simulink model "Rider_Controls_ControlHarness"  (R2014b)
settings: configuration reference "Embedded_Configuration" (kept outside this file)
PostLoadFcn:
  | load('Embedded_Config.mat')
model workspace: external: MAT-File C:\Users\Sean\Desktop\Buckeye Current\MagicSimNode\Rider_Controls.mat (data not in the file)
undefined symbols (not defined in the file or in its folder): canChannel, sigbuilder_block
libraries: canlib x10, canmsglib x8, dspswit3 x2, simulink x1, realtime_pacer_lib x1, dspsigattribs x1
settings Model: Creator=The MathWorks Inc.  LastModifiedBy=Sean

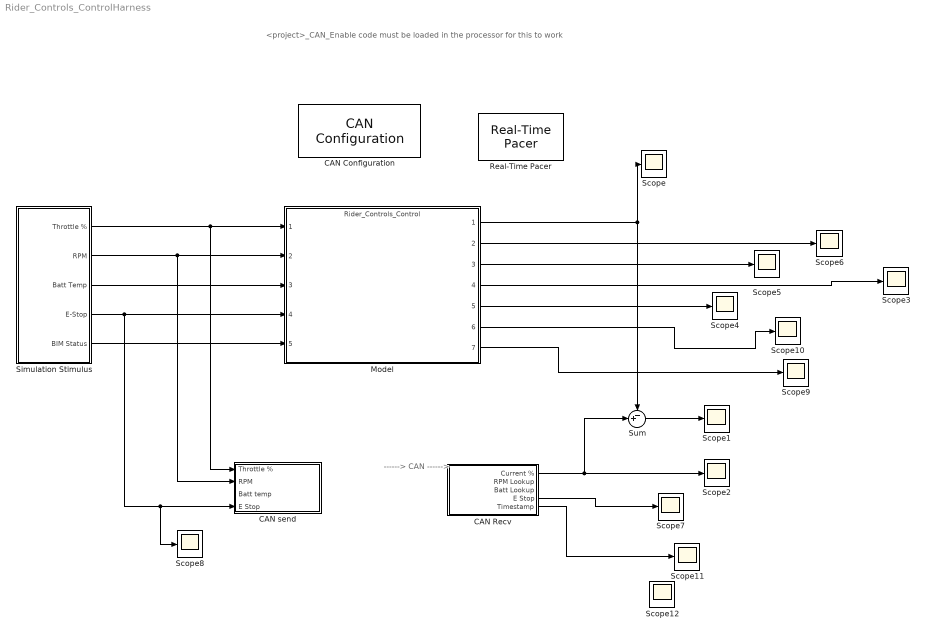
== system Rider_Controls_ControlHarness ==
  note: <project>_CAN_Enable code must be loaded
      | in the processor for this to work
  note: ------> CAN ------>
  CAN Configuration : canlib/CAN Configuration  BlockHandle=3197.0009  DeviceMenu=Kvaser Virtual 1 (Channel 1)  Device=Kvaser Eagle 1 (Channel 1)  ObjConstructor=canChannel('Kvaser', 'Eagle 1', 1)  BusSpeed=500000  EnableBitParameters=off  SJW=1  TSEG1=4  TSEG2=3  NSamples=1  AckMode=Normal
  CAN Recv : Subsystem
  CAN send : Subsystem
  Model : ModelReference  ModelNameDialog=Rider_Controls_Control.slx  SimulationMode=Normal  ModelReferenceVersion=1.163  CopyOfModelName=Rider_Controls_Control.slx  DefaultDataLogging=on
  Real-Time Pacer : realtime_pacer_lib/Real-Time Pacer  simTimePerRealTime=1
  Scope{,1..12} (13 alike) : Scope
      Scope settings: YMin=-0.2  YMax=1.2
      Scope10 settings: SaveName=ScopeData10
      Scope11 settings: TimeRange=20  SaveName=ScopeData11
      Scope12 settings: TimeRange=10  YMin=0  YMax=4  SaveName=ScopeData12
      Scope2 settings: TimeRange=10  SaveName=ScopeData2
      Scope3 settings: SaveName=ScopeData3
      Scope4 settings: SaveName=ScopeData4
      Scope5 settings: YMin=-0.2  YMax=1.2  SaveName=ScopeData5
      Scope6 settings: YMin=-0.2  YMax=1.2  SaveName=ScopeData6
      Scope7 settings: TimeRange=10  SaveName=ScopeData7
      Scope8 settings: TimeRange=10  SaveName=ScopeData8
      Scope9 settings: SaveName=ScopeData9
  Simulation Stimulus : Subsystem
  Sum : Sum  Inputs=-+|
  wires:
  CAN Recv/1(Current %) -> Sum/2, Scope2/1
  Sum/1 -> Scope1/1
  Simulation Stimulus/1("Throttle % ") -> CAN send/1(Throttle %), Model/1
  Simulation Stimulus/2(RPM) -> CAN send/2(RPM), Model/2
  Simulation Stimulus/3(Batt Temp) -> Model/3
  Model/1 -> Sum/1, Scope/1
  Model/4 -> Scope3/1
  Model/5 -> Scope4/1
  Model/2 -> Scope6/1
  Model/3 -> Scope5/1
  Simulation Stimulus/4(E-Stop) -> Scope8/1, CAN send/4(E Stop), Model/4
  CAN Recv/4(E Stop) -> Scope7/1
  Model/7 -> Scope9/1
  Simulation Stimulus/5(BIM Status) -> Model/5
  Model/6 -> Scope10/1
  CAN Recv/5(Timestamp) -> Scope11/1
  ? -> Scope12/1

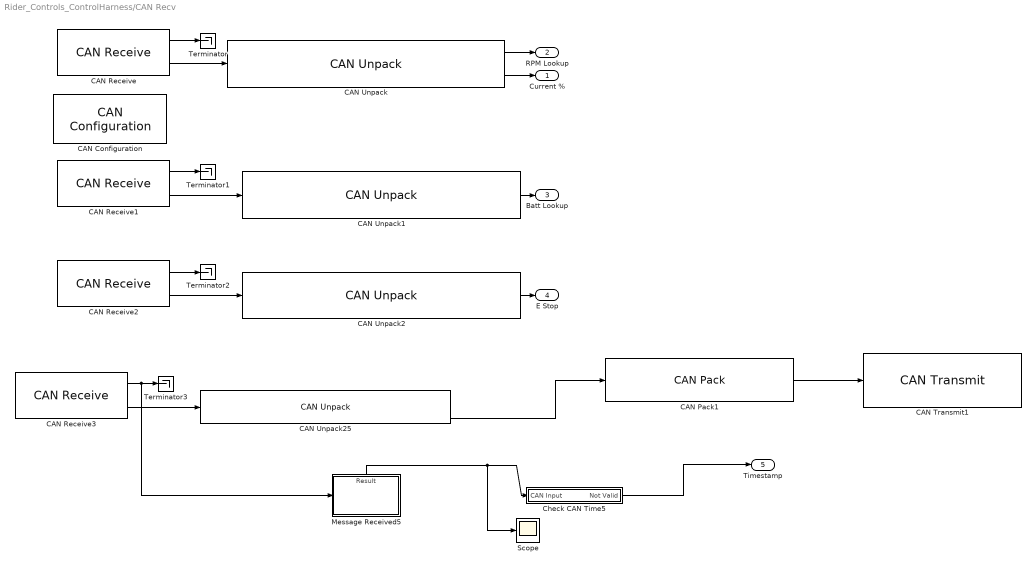
== system Rider_Controls_ControlHarness/CAN Recv ==
  CAN Configuration : canlib/CAN Configuration  BlockHandle=3204.0009  DeviceMenu=Kvaser Virtual 1 (Channel 1)  Device=Kvaser Virtual 1 (Channel 1)  ObjConstructor=canChannel('Kvaser', 'Virtual 1', 1)  BusSpeed=500000  EnableBitParameters=off  SJW=1  TSEG1=4  TSEG2=3  NSamples=1  AckMode=Normal
  CAN Pack1 : canmsglib/CAN Pack  CANdbFile=C:\Users\Nathan\Desktop\Git\EmbeddedCoderC2000\Rider_Controls\Rider_Controls_Debug.dbc  MsgList=Control_Input3  MsgName=Control_Input3  MsgIDType=Standard (11-bit identifier)  MsgIdentifier=2  MsgLength=8  SignalInfo=Batt_Temp$0$32$1$3$1$0$1$0$-10000$10000$#  NSignals=1  StartBits=str2num('[int32(0)]')  SignalSizes=str2num('[int32(32)]')  ByteOrders=str2num('[int32(1)]')  DataTypes=str2num('[int32(3)]')  MultiplexTypes=str2num('[int32(1)]')  MultiplexValues=str2num('[double(0)]')  Factors=str2num('[double(1)]')  Offsets=str2num('[double(0)]')  Minimums=str2num('[double(-10000)]')  Maximums=str2num('[double(10000)]')  Remote=off
      settings: DataFormat=CANdb specified signals
  CAN Receive : canlib/CAN Receive  BlockHandle=3206.0009  DeviceMenu=Kvaser Virtual 1 (Channel 1)  Device=Kvaser Eagle 1 (Channel 1)  ObjConstructor=canChannel('Kvaser', 'Eagle 1', 1)  EnableStandardIDsFilter=off  StandardIDs=1  EnableExtendedIDsFilter=off  ExtendedIDs=0  SampleTime=.01  MsgsPerTimestep=all  StdIDsCombo=Allow only  ExtIDsCombo=Block all  InternalFilterUpdateStatus=on
  CAN Receive1 : canlib/CAN Receive  BlockHandle=3207.0009  DeviceMenu=Kvaser Virtual 1 (Channel 1)  Device=Kvaser Eagle 1 (Channel 1)  ObjConstructor=canChannel('Kvaser', 'Eagle 1', 1)  EnableStandardIDsFilter=off  StandardIDs=3  EnableExtendedIDsFilter=off  ExtendedIDs=0  SampleTime=.01  MsgsPerTimestep=all  StdIDsCombo=Allow only  ExtIDsCombo=Block all  InternalFilterUpdateStatus=on
  CAN Receive2 : canlib/CAN Receive  BlockHandle=4510.0004  DeviceMenu=Kvaser Virtual 1 (Channel 1)  Device=Kvaser Eagle 1 (Channel 1)  ObjConstructor=canChannel('Kvaser', 'Eagle 1', 1)  EnableStandardIDsFilter=off  StandardIDs=5  EnableExtendedIDsFilter=off  ExtendedIDs=0  SampleTime=.01  MsgsPerTimestep=all  StdIDsCombo=Allow only  ExtIDsCombo=Block all  InternalFilterUpdateStatus=on
  CAN Receive3 : canlib/CAN Receive  BlockHandle=4511.0004  DeviceMenu=Kvaser Eagle 1 (Channel 1)  Device=Kvaser Eagle 1 (Channel 1)  ObjConstructor=canChannel('Kvaser', 'Eagle 1', 1)  EnableStandardIDsFilter=off  StandardIDs=831  EnableExtendedIDsFilter=off  ExtendedIDs=0  SampleTime=.5  MsgsPerTimestep=all  StdIDsCombo=Allow only  ExtIDsCombo=Block all  InternalFilterUpdateStatus=on
  CAN Transmit1 : canlib/CAN Transmit  BlockHandle=4512.0004  DeviceMenu=Kvaser Virtual 1 (Channel 1)  Device=Kvaser Eagle 1 (Channel 1)  ObjConstructor=canChannel('Kvaser', 'Eagle 1', 1)  EnablePeriodicTransmit=on  MessagePeriod=.01
  CAN Unpack : canmsglib/CAN Unpack  CANdbFile=C:\Users\Nathan\Desktop\Git\EmbeddedCoderC2000\Rider_Controls\Rider_Controls_Debug.dbc  MsgList=Control_Ouput  MsgName=Control_Ouput  MsgIDType=Standard (11-bit identifier)  MsgIdentifier=1  MsgLength=8  SignalInfo=Lookup$32$32$1$3$1$0$1$0$-10000$10000$#Motor_Current_percent$0$32$1$3$1$0$1$0$-1000$1000$#  NSignals=2  IDPort=off  TimestampPort=off  ErrorPort=off  RemotePort=off  LengthPort=off  StatusPort=off  StartBits=str2num('[int32(32);int32(0)]')  SignalSizes=str2num('[int32(32);int32(32)]')  ByteOrders=str2num('[int32(1);int32(1)]')  DataTypes=str2num('[int32(3);int32(3)]')  MultiplexTypes=str2num('[int32(1);int32(1)]')  MultiplexValues=str2num('[double(0);double(0)]')  Factors=str2num('[double(1);double(1)]')  Offsets=str2num('[double(0);double(0)]')  Minimums=str2num('[double(-10000);double(-1000)]')  Maximums=str2num('[double(10000);double(1000)]')
      settings: DataFormat=CANdb specified signals
  CAN Unpack1 : canmsglib/CAN Unpack  CANdbFile=C:\Users\Nathan\Desktop\Git\EmbeddedCoderC2000\Rider_Controls\Rider_Controls_Debug.dbc  MsgList=Control_Output3  MsgName=Control_Output3  MsgIDType=Standard (11-bit identifier)  MsgIdentifier=3  MsgLength=8  SignalInfo=Batt_Lookup$0$32$1$3$1$0$1$0$-1000$10000$#  NSignals=1  IDPort=off  TimestampPort=off  ErrorPort=off  RemotePort=off  LengthPort=off  StatusPort=off  StartBits=str2num('[int32(0)]')  SignalSizes=str2num('[int32(32)]')  ByteOrders=str2num('[int32(1)]')  DataTypes=str2num('[int32(3)]')  MultiplexTypes=str2num('[int32(1)]')  MultiplexValues=str2num('[double(0)]')  Factors=str2num('[double(1)]')  Offsets=str2num('[double(0)]')  Minimums=str2num('[double(-1000)]')  Maximums=str2num('[double(10000)]')
      settings: DataFormat=CANdb specified signals
  CAN Unpack2 : canmsglib/CAN Unpack  CANdbFile=C:\Users\Nathan\Desktop\Git\EmbeddedCoderC2000\Rider_Controls\Rider_Controls_Debug.dbc  MsgList=Control_Output4  MsgName=Control_Output4  MsgIDType=Standard (11-bit identifier)  MsgIdentifier=5  MsgLength=8  SignalInfo=EStop$0$32$1$3$1$0$1$0$-Inf$Inf$#  NSignals=1  IDPort=off  TimestampPort=off  ErrorPort=off  RemotePort=off  LengthPort=off  StatusPort=off  StartBits=str2num('[int32(0)]')  SignalSizes=str2num('[int32(32)]')  ByteOrders=str2num('[int32(1)]')  DataTypes=str2num('[int32(3)]')  MultiplexTypes=str2num('[int32(1)]')  MultiplexValues=str2num('[double(0)]')  Factors=str2num('[double(1)]')  Offsets=str2num('[double(0)]')  Minimums=str2num('[double(-Inf)]')  Maximums=str2num('[double(Inf)]')
      settings: DataFormat=CANdb specified signals
  CAN Unpack25 : canmsglib/CAN Unpack  CANdbFile=C:\Users\Sean\Desktop\Buckeye Current\Databases\RW3.dbc  MsgList=CellTemp20  MsgName=CellTemp20  MsgIDType=Standard (11-bit identifier)  MsgIdentifier=831  MsgLength=8  SignalInfo=CellTemp39$0$32$1$3$1$0$1$0$-Inf$Inf$#CellTemp40$32$32$1$3$1$0$1$0$-Inf$Inf$#  NSignals=2  IDPort=off  TimestampPort=on  ErrorPort=off  RemotePort=off  LengthPort=off  StatusPort=off  StartBits=str2num('[int32(0);int32(32)]')  SignalSizes=str2num('[int32(32);int32(32)]')  ByteOrders=str2num('[int32(1);int32(1)]')  DataTypes=str2num('[int32(3);int32(3)]')  MultiplexTypes=str2num('[int32(1);int32(1)]')  MultiplexValues=str2num('[double(0);double(0)]')  Factors=str2num('[double(1);double(1)]')  Offsets=str2num('[double(0);double(0)]')  Minimums=str2num('[double(-Inf);double(-Inf)]')  Maximums=str2num('[double(Inf);double(Inf)]')
      settings: DataFormat=CANdb specified signals
  Check CAN Time5 : Subsystem
  Message Received5 : Subsystem  TreatAsAtomicUnit=on
  Scope : Scope
      settings: YMin=0  YMax=20  SaveName=ScopeData14
  Terminator{,1..3} (4 alike) : Terminator
  Current % : Outport
  RPM Lookup : Outport  Port=2
  Batt Lookup : Outport  Port=3
  E Stop : Outport  Port=4
  Timestamp : Outport  Port=5
  wires:
  CAN Receive/1 -> Terminator/1
  CAN Receive/2 -> CAN Unpack/1
  CAN Unpack/2 -> Current %/1
  CAN Unpack/1 -> RPM Lookup/1
  CAN Receive1/1 -> Terminator1/1
  CAN Receive1/2 -> CAN Unpack1/1
  CAN Unpack1/1 -> Batt Lookup/1
  CAN Receive2/1 -> Terminator2/1
  CAN Receive2/2 -> CAN Unpack2/1
  CAN Unpack2/1 -> E Stop/1
  CAN Receive3/2 -> CAN Unpack25/1
  CAN Receive3/1 -> Message Received5/Trigger, Terminator3/1
  CAN Unpack25/3 -> CAN Pack1/1
  CAN Pack1/1 -> CAN Transmit1/1
  Message Received5/1(Result) -> Scope/1, Check CAN Time5/1(CAN Input)
  Check CAN Time5/1(Not Valid) -> Timestamp/1

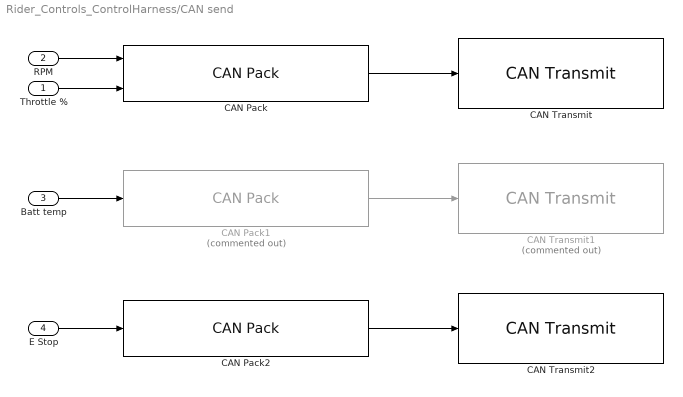
== system Rider_Controls_ControlHarness/CAN send ==
  Throttle % : Inport  OutDataTypeStr=single
  RPM : Inport  Port=2  OutDataTypeStr=single
  Batt temp : Inport  Port=3  OutDataTypeStr=single
  E Stop : Inport  Port=4
  CAN Pack : canmsglib/CAN Pack  CANdbFile=C:\Users\Nathan\Desktop\Git\EmbeddedCoderC2000\Rider_Controls\Rider_Controls_Debug.dbc  MsgList=Control_Input  MsgName=Control_Input12  MsgIDType=Standard (11-bit identifier)  MsgIdentifier=0  MsgLength=8  SignalInfo=RPM$32$32$1$3$1$0$1$0$-100000$100000$#Throttle$0$32$1$3$1$0$1$0$-1000$1000$#  NSignals=2  StartBits=str2num('[int32(32);int32(0)]')  SignalSizes=str2num('[int32(32);int32(32)]')  ByteOrders=str2num('[int32(1);int32(1)]')  DataTypes=str2num('[int32(3);int32(3)]')  MultiplexTypes=str2num('[int32(1);int32(1)]')  MultiplexValues=str2num('[double(0);double(0)]')  Factors=str2num('[double(1);double(1)]')  Offsets=str2num('[double(0);double(0)]')  Minimums=str2num('[double(-100000);double(-1000)]')  Maximums=str2num('[double(100000);double(1000)]')  Remote=off
      settings: DataFormat=CANdb specified signals
  CAN Pack1 : canmsglib/CAN Pack  Commented=on  CANdbFile=C:\Users\Nathan\Desktop\Git\EmbeddedCoderC2000\Rider_Controls\Rider_Controls_Debug.dbc  MsgList=Control_Input3  MsgName=Control_Input3  MsgIDType=Standard (11-bit identifier)  MsgIdentifier=2  MsgLength=8  SignalInfo=Batt_Temp$0$32$1$3$1$0$1$0$-10000$10000$#  NSignals=1  StartBits=str2num('[int32(0)]')  SignalSizes=str2num('[int32(32)]')  ByteOrders=str2num('[int32(1)]')  DataTypes=str2num('[int32(3)]')  MultiplexTypes=str2num('[int32(1)]')  MultiplexValues=str2num('[double(0)]')  Factors=str2num('[double(1)]')  Offsets=str2num('[double(0)]')  Minimums=str2num('[double(-10000)]')  Maximums=str2num('[double(10000)]')  Remote=off
      settings: DataFormat=CANdb specified signals
  CAN Pack2 : canmsglib/CAN Pack  CANdbFile=C:\Users\Nathan\Desktop\Git\EmbeddedCoderC2000\Rider_Controls\Rider_Controls_Debug.dbc  MsgList=Control_Input4  MsgName=Control_Input4  MsgIDType=Standard (11-bit identifier)  MsgIdentifier=4  MsgLength=8  SignalInfo=EStop$0$32$1$2$1$0$1$0$-Inf$Inf$#  NSignals=1  StartBits=str2num('[int32(0)]')  SignalSizes=str2num('[int32(32)]')  ByteOrders=str2num('[int32(1)]')  DataTypes=str2num('[int32(2)]')  MultiplexTypes=str2num('[int32(1)]')  MultiplexValues=str2num('[double(0)]')  Factors=str2num('[double(1)]')  Offsets=str2num('[double(0)]')  Minimums=str2num('[double(-Inf)]')  Maximums=str2num('[double(Inf)]')  Remote=off
      settings: DataFormat=CANdb specified signals
  CAN Transmit : canlib/CAN Transmit  BlockHandle=4565.0001  DeviceMenu=Kvaser Virtual 1 (Channel 1)  Device=Kvaser Eagle 1 (Channel 1)  ObjConstructor=canChannel('Kvaser', 'Eagle 1', 1)  EnablePeriodicTransmit=on  MessagePeriod=.01
  CAN Transmit1 : canlib/CAN Transmit  Commented=on  BlockHandle=4566.0001  DeviceMenu=Kvaser Virtual 1 (Channel 1)  Device=Kvaser Eagle 1 (Channel 1)  ObjConstructor=canChannel('Kvaser', 'Eagle 1', 1)  EnablePeriodicTransmit=on  MessagePeriod=.01
  CAN Transmit2 : canlib/CAN Transmit  BlockHandle=4567.0001  DeviceMenu=Kvaser Virtual 1 (Channel 1)  Device=Kvaser Eagle 1 (Channel 1)  ObjConstructor=canChannel('Kvaser', 'Eagle 1', 1)  EnablePeriodicTransmit=on  MessagePeriod=.01
  wires:
  CAN Pack/1 -> CAN Transmit/1
  RPM/1 -> CAN Pack/1
  Throttle %/1 -> CAN Pack/2
  Batt temp/1 -> CAN Pack1/1
  CAN Pack1/1 -> CAN Transmit1/1
  E Stop/1 -> CAN Pack2/1
  CAN Pack2/1 -> CAN Transmit2/1

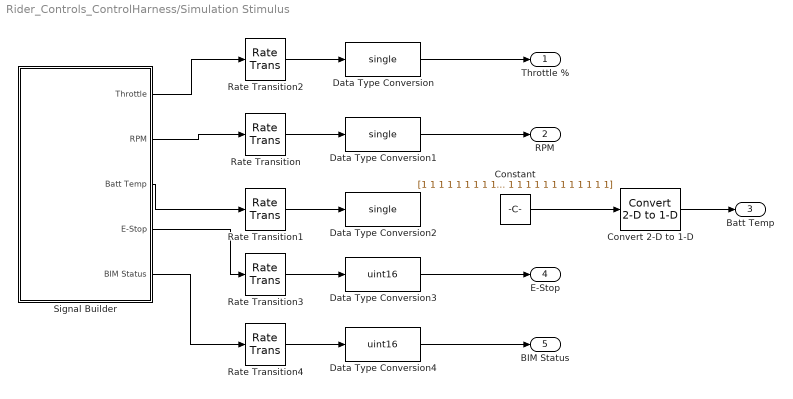
== system Rider_Controls_ControlHarness/Simulation Stimulus ==
  Constant : Constant  Value=[1 1 1 1 1 1 1 1 1 1 1 1 1 1 1 1 1 1 1 1 1 1 1 1 1 1 1 1 1 1 1 1 1 1 1 1 1 1 1 1]  VectorParams1D=off  OutDataTypeStr=single
  Convert 2-D to 1-D : dspsigattribs/Convert 2-D to 1-D
  Data Type Conversion : DataTypeConversion  OutDataTypeStr=single  RndMeth=Simplest
  Data Type Conversion1 : DataTypeConversion  OutDataTypeStr=single  RndMeth=Simplest
  Data Type Conversion2 : DataTypeConversion  OutDataTypeStr=single  RndMeth=Simplest
  Data Type Conversion3 : DataTypeConversion  OutDataTypeStr=uint16  RndMeth=Simplest
  Data Type Conversion4 : DataTypeConversion  OutDataTypeStr=uint16  RndMeth=Simplest
  Rate Transition{,1..4} (5 alike) : RateTransition  OutPortSampleTime=.01
  Signal Builder : Subsystem  Tag=STV Subsys  LoadFcn=sigbuilder_block('load');  StartFcn=sigbuilder_block('start');  StopFcn=sigbuilder_block('stop');  ClipboardFcn=sigbuilder_block('clipboard');  mask(Sigbuilder block){}
      mask help: Simulink:masks:SigbuilderBlock_MD
      mask init:
      | if ~strcmp(get_param(bdroot(gcbh),'SimulationStatus'),'stopped') tuvar = sigbuilder_block('maskInit'); end
      settings: CopyFcn=sigbuilder_block('copy');  DeleteFcn=sigbuilder_block('delete');  ModelCloseFcn=sigbuilder_block('modelClose');  PreSaveFcn=sigbuilder_block('preSave');  PauseFcn=sigbuilder_block('pause');  ContinueFcn=sigbuilder_block('continue');  NameChangeFcn=sigbuilder_block('namechange');  OpenFcn=sigbuilder_block('open',[437.6 199.2 550.4 400 ]);  CloseFcn=sigbuilder_block('close');
      mask Display: plot(0, 0, 100, 100,[2, 2, 32, 32, 2], [68, 8, 8, 68, 68],[32, 2], [38, 38], [32, 19, 2],[53, 60, 44], [32, 17, 17, 2],[16, 16, 31, 31]);txt = getActiveGroup(gcbh);text(2, 100, txt,'verticalAlignment', 'top');
  "Throttle % " : Outport  OutDataTypeStr=single
  RPM : Outport  Port=2  OutDataTypeStr=single
  Batt Temp : Outport  Port=3  OutDataTypeStr=single
  E-Stop : Outport  Port=4
  BIM Status : Outport  Port=5
  wires:
  Rate Transition/1 -> Data Type Conversion1/1
  Signal Builder/2(RPM) -> Rate Transition/1
  Signal Builder/3(Batt Temp) -> Rate Transition1/1
  Rate Transition1/1 -> Data Type Conversion2/1
  Rate Transition2/1 -> Data Type Conversion/1
  Data Type Conversion/1 -> "Throttle % "/1
  Data Type Conversion1/1 -> RPM/1
  Signal Builder/1(Throttle) -> Rate Transition2/1
  Signal Builder/4(E-Stop) -> Rate Transition3/1
  Rate Transition3/1 -> Data Type Conversion3/1
  Data Type Conversion3/1 -> E-Stop/1
  Signal Builder/5(BIM Status) -> Rate Transition4/1
  Rate Transition4/1 -> Data Type Conversion4/1
  Data Type Conversion4/1 -> BIM Status/1
  Constant/1 -> Convert 2-D to 1-D/1
  Convert 2-D to 1-D/1 -> Batt Temp/1

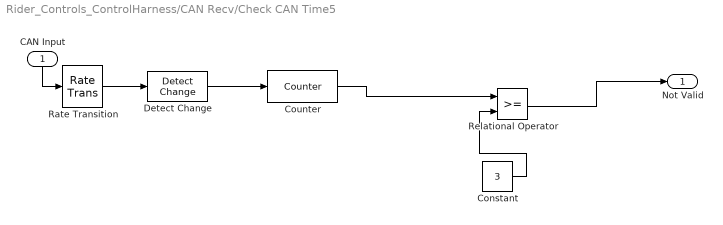
== system Rider_Controls_ControlHarness/CAN Recv/Check CAN Time5 ==
  CAN Input : Inport
  Constant : Constant  Value=3
  Counter : dspswit3/Counter  Direction=Up  CountEvent=Free running  CounterSize=16 bits  MaxCount=255  InitialCount=0  Output=Count  HitValue=1  ResetInput=on  SamplesPerFrame=1  Ts=1  CntDtype=uint16  HitDtype=Logical
  Detect Change : simulink/Logic and Bit Operations/Detect Change  vinit=0  InputProcessing=Inherited  OutDataTypeStr=boolean
  Rate Transition : RateTransition  X0=1  OutPortSampleTime=1
  Relational Operator : RelationalOperator  OutDataTypeStr=boolean
  Not Valid : Outport
  wires:
  CAN Input/1 -> Rate Transition/1
  Relational Operator/1 -> Not Valid/1
  Counter/1 -> Relational Operator/1
  Constant/1 -> Relational Operator/2
  Rate Transition/1 -> Detect Change/1
  Detect Change/1 -> Counter/1

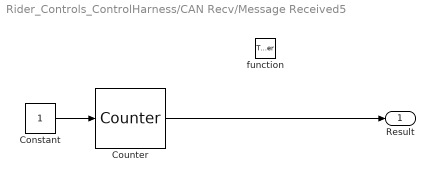
== system Rider_Controls_ControlHarness/CAN Recv/Message Received5 ==
  function : TriggerPort  TriggerType=function-call
  Constant : Constant
  Counter : dspswit3/Counter  Direction=Up  CountEvent=Non-zero sample  CounterSize=16 bits  MaxCount=255  InitialCount=0  Output=Count  HitValue=32  ResetInput=off  SamplesPerFrame=1  Ts=-1  CntDtype=uint16  HitDtype=Logical
  Result : Outport  OutputWhenDisabled=reset  InitialOutput=0
  wires:
  Counter/1 -> Result/1
  Constant/1 -> Counter/1

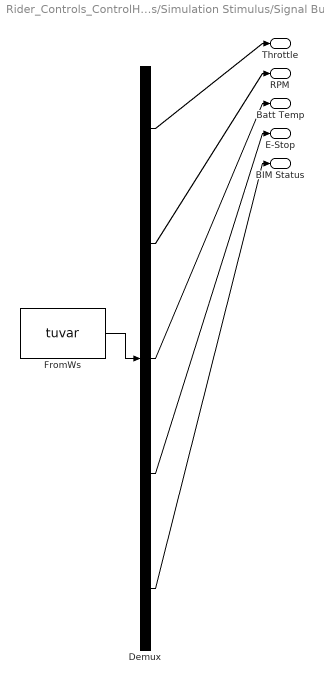
== system Rider_Controls_ControlHarness/Simulation Stimulus/Signal Builder ==
  Demux : Demux  Tag=STV Demux  Outputs=5
  FromWs : FromWorkspace  Tag=STV FromWs  VariableName=tuvar  SampleTime=0
      SigBuilderData=|
      | common.afterFinalStr = 'Extrapolate'
      | common.sampleTime = 0
      | dataSet.timeRange = [0 10]
      | dataSet.name = 'Group 1'
      | sbobj.Groups.Name = 'Group 1'
      | sbobj.Groups.Signals(1).Name = 'Throttle'
      | sbobj.Groups.Signals(1).XData = [0 3.7 3.7 7.26 7.26 10]
      | sbobj.Groups.Signals(1).YData = [0.81 0.81 0.26 0.26 0.11 0.11]
      | sbobj.Groups.Signals(2).Name = 'RPM'
      | sbobj.Groups.Signals(2).XData = [0 3 6.02 10]
      | sbobj.Groups.Signals(2).YData = [0 0 0 4000]
      | sbobj.Groups.Signals(3).Name = 'Batt Temp'
      | sbobj.Groups.Signals(3).XData = [0 3 6 6 10]
      | sbobj.Groups.Signals(3).YData = [0 0 100 0 100]
      | sbobj.Groups.Signals(4).Name = 'E-Stop'
      | sbobj.Groups.Signals(4).XData = [0 1.78 1.78 3.62 3.62 10]
      | sbobj.Groups.Signals(4).YData = [0 0 1 1 0 0]
      | sbobj.Groups.Signals(5).Name = 'BIM Status'
      | sbobj.Groups.Signals(5).XData = [0 4 4 4.3 4.3 10]
      | sbobj.Groups.Signals(5).YData = [0 0 1 1 0 0]
  Throttle : Outport  Tag=STV Outport
  RPM : Outport  Tag=STV Outport  Port=2
  Batt Temp : Outport  Tag=STV Outport  Port=3
  E-Stop : Outport  Tag=STV Outport  Port=4
  BIM Status : Outport  Tag=STV Outport  Port=5
  wires:
  FromWs/1 -> Demux/1
  Demux/1 -> Throttle/1
  Demux/2 -> RPM/1
  Demux/3 -> Batt Temp/1
  Demux/4 -> E-Stop/1
  Demux/5 -> BIM Status/1
